simulink model "Simple_Variable_PID_KNN_gain_selector"  (R2020a)
settings: Solver=VariableStepAuto  StartTime=0.0  StopTime=0.08  RelTol=1e-3
undefined symbols (not defined in the file): Ion, Lithium
libraries: powerlib x15, simulink x3, powerlib_meascontrol x3, eeStairGenerator x3, electricdrivelib x1, re_lib x1
settings Model: Creator=Javier  LastModifiedBy=Javier

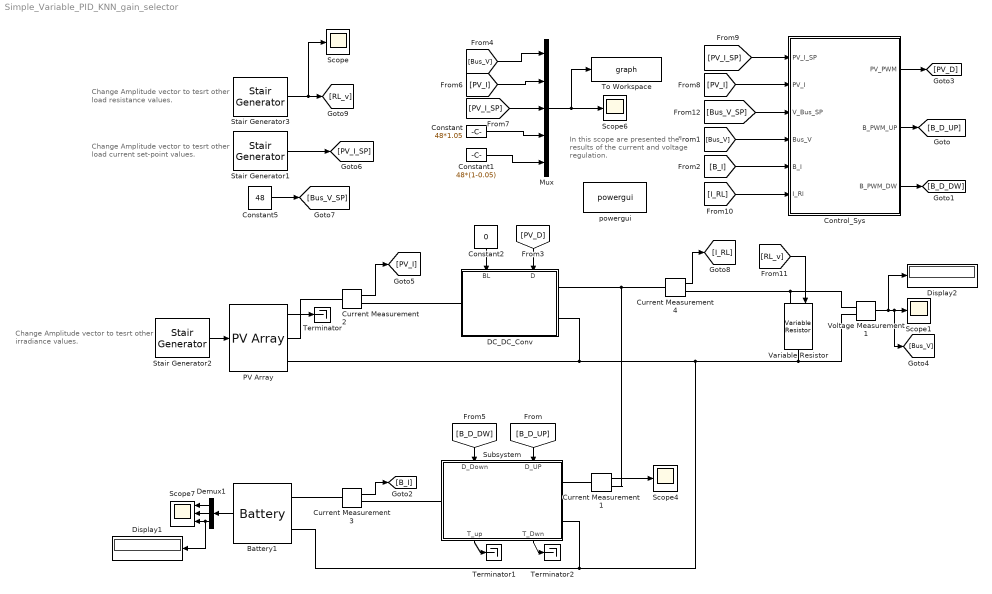
== system Simple_Variable_PID_KNN_gain_selector ==
  note: In this scope are presented the
      | results of the current and voltage
      | regulation.
  note: Change Amplitude vector to tesrt other
      | load resistance values.
  note: Change Amplitude vector to tesrt other
      | load current set-point values.
  note: Change Amplitude vector to tesrt other
      | irradiance values.
  Battery1 : electricdrivelib/Extra Sources/Battery  BatType=Lithium-Ion  ShowTempParam=off  ThermalPreset=no  ShowAgeParam=off  NomV=38.4  NomQ=2500  SOC=60  Batt_Tr=30  PresetModel=on  MaxQ=2500  MinV=28.8  FullV=44.6971  Dis_rate=1086.9565  R=0.0001536  Normal_OP=2260.8696  expZone="[41.48682      122.8261]"  current=[6.5 13 32.5]  Units=Time  Tci=20  NomT=20  T2=-30  MaxQ2=4.8  FullV2=7.1  Normal_OP2=5.655  expZone2="[6.58           1]"  Rca=0.6  ti=2000  Dp=0  Neq0=0  Tsim=1e6  Ta1=25  Qeol=5.4*0.9  Reol=0.013333*1.2  Char_age=[2.3478, 3]  Dis_age=[2.3478, 10]  N1=1500  N2=10500  N3=1000  N4=1400  Ta2=45  N5=950
  Constant : Constant  Value=48*1.05
  Constant1 : Constant  Value=48*(1-0.05)
  Constant2 : Constant  Value=0
  Constant5 : Constant  Value=48
  Control_Sys : Subsystem
  Current Measurement{1..4} (4 alike) : powerlib/Measurements/Current Measurement  PhasorSimulation=off  OutputType=Complex  PSBequivalent=0
  DC_DC_Conv : Subsystem
      settings: PortSchema="{\"entries\":[{\"content\":{\"sides\":[{\"content\":{\"connectorIds\":[\"LConn1\"]},\"type\":\"ConnectorPlacement.EquallySpacedRectSide\",\"uuid\":\"00f7090b-60ae-413e-b809-f771630d6751\"},{\"content\":{\"connectorIds\":[\"RConn1\",\"RConn2\"],\"side\":\"RIGHT\"},\"type\":\"ConnectorPlacement.EquallySpacedRectSide\",\"uuid\":\"f0025ab7-a9d8-466a-8e23-704d013948c1\"},{\"content\":{\"connectorIds\":[\"In1\",\"In2\"],\"side\":\"TOP\"},\"type\":\"ConnectorPlacement.EquallySpacedRectSide\",\"uuid\":\"5a345099-75bf-400d-9bb3-22f689fa92ef\"}]},\"type\":\"ConnectorPlacement.EquallySpacedConnector\",\"uuid\":\"2e1b2c5d-1adb-4779-83d3-3c40793dd951\"}],\"packageUris\":[\"http://schema.mathworks.com/mf0/Connector/19700101\"],\"version\":\"1.0\"}"
  Demux1 : Demux  Outputs=3
  Display1 : Display
  Display2 : Display
  Mux : Mux  Inputs=5
  PV Array : re_lib/Solar/PV Array  Npar=7  Nser=1  PlotType=array @ 1000 W/m2 & specified temperatures  S_vec="[ 1000  500  100 ]"  Temp_C_vec="[ 45 25  ]"  ModuleName=LG Electronics LG300N1W-G3  PlotWhenSelected=off  Pm=302.72  Ncell=60  Voc=39.5  Isc=10.05  Vm=32  Im=9.46  beta_Voc_pc=-0.3  alpha_Isc_pc=0.03  beta_Voc=-0.1185  alpha_Isc=0.003015  IL=10.0926  I0=3.3235e-11  nI=0.96984  Rsh=212.8143  Rs=0.31448  RobustModel=on  RobustCellTemperature=25  BAL=on  Tc=1e-7  Tfilter=1e-8
  Scope{,1,4,6} (4 alike) : Scope
  Scope7 : Scope  NumInputPorts=3
  Stair Generator1 : eeStairGenerator/Stair Generator  LabelModeActiveChoice=Discrete  TimeInput=[0 1 2 3 4 5 6]*0.01  AmplitudeInput=[0 3.323 6.645 49.65 23.28 6.645 0]  SampleTime=1/(1000e3)  RepeatPattern=off  OutDataTypeStr=double
      settings: SourceProductBaseCode=PS
  Stair Generator2 : eeStairGenerator/Stair Generator  LabelModeActiveChoice=Discrete  TimeInput=[0 1 2 3 4 5 6]*0.01  AmplitudeInput=[0 50 100 750 350 100 0]  SampleTime=1/(1000e3)  RepeatPattern=off  OutDataTypeStr=double
      settings: SourceProductBaseCode=PS
  Stair Generator3 : eeStairGenerator/Stair Generator  LabelModeActiveChoice=Discrete  TimeInput=[0 1 2 3 4 5 6]*0.01  AmplitudeInput=[10 5 1 10 20 20 20]  SampleTime=1/(1000e3)  RepeatPattern=off  OutDataTypeStr=double
      settings: SourceProductBaseCode=PS
  Subsystem : Subsystem
      settings: PortSchema="{\"entries\":[{\"content\":{\"sides\":[{\"content\":{\"connectorIds\":[\"LConn1\"]},\"type\":\"ConnectorPlacement.EquallySpacedRectSide\",\"uuid\":\"a9530ab3-8980-4dba-8483-d408c1c24a59\"},{\"content\":{\"connectorIds\":[\"RConn1\",\"RConn2\"],\"side\":\"RIGHT\"},\"type\":\"ConnectorPlacement.EquallySpacedRectSide\",\"uuid\":\"f691113d-6eb3-43ec-a6a4-3d8fb6884df6\"},{\"content\":{\"connectorIds\":[\"In1\",\"In2\"],\"side\":\"TOP\"},\"type\":\"ConnectorPlacement.EquallySpacedRectSide\",\"uuid\":\"a9eb11b6-05d7-4dbc-be9d-a17fd8550bb3\"},{\"content\":{\"connectorIds\":[\"Out1\",\"Out2\"],\"side\":\"BOTTOM\"},\"type\":\"ConnectorPlacement.EquallySpacedRectSide\",\"uuid\":\"90c7147c-e357-433a-9063-3b2a71587c45\"}]},\"type\":\"ConnectorPlacement.EquallySpacedConnector\",\"uuid\":\"b290d60f-d8ab-41f4-904b-2a909013e95d\"}],\"packageUris\":[\"http://schema.mathworks.com/mf0/Connector/19700101\"],\"version\":\"1.0\"}"
  Terminator : Terminator
  Terminator1 : Terminator
  Terminator2 : Terminator
  To Workspace : ToWorkspace  VariableName=graph  SaveFormat=Timeseries  SampleTime=-1
  Variable Resistor : powerlib/Elements/Variable Resistor  Rabsmin=1e-3
      settings: SourceProductBaseCode=PS
  Voltage Measurement1 : powerlib/Measurements/Voltage Measurement  PhasorSimulation=off  OutputType=Complex  PSBequivalent=0
  powergui : powerlib/powergui  Priority=1  SimulationMode=Discrete  SampleTime=1/(1000e3)  frequency=60  Iterations=50  frequencyindice=0  Pbase=100e6  ErrMax=1e-4  UnitsV=kV  UnitsW=MW  buscounter=0  FunctionMessages=off  echomessages=off  EnableUseOfTLC=off  CurrentSourceSwitches=off  DisableSnubberDevices=off  DisableRonSwitches=off  DisableVfSwitches=off  DisplayEquations=off  AutomaticDiscreteSolvers=off  SolverType=Tustin/Backward Euler (TBE)  Interpol=off  ExternalGateDelay=off  methode=off  Ts=100  x0status=blocks  SPID=on  SwTol=0  HookPort=off  NonlinearTolerance=1e-4  nMaxIteration=100  ContinueOnMaxIteration=off  RestoreLinks=warning  ResistiveCurrentMeasurement=off  Frange=[0:2:500]  Ylog=off  Xlog=on  ShowGrid=off  save=off  variable=ZData  structure=0  ZoomFFT=off  StartTime=0.0  cycles=1  DisplayStyle=1  fundamental=60  FreqAxis=off  MaxFrequency=1000  frequencyindicesteady=1  RmsSteady=1  display=off
  wires:
  Current Measurement2/1 -> [PV_I]
  Mux/1 -> To Workspace/1, Scope6/1
  Constant2/1 -> DC_DC_Conv/1(BL)
  Demux1/2 -> Scope7/2
  Demux1/3 -> Display1/1, Scope7/3
  Demux1/1 -> Scope7/1
  Battery1/1 -> Demux1/1
  Voltage Measurement1/1 -> [Bus_V], Scope1/1, Display2/1
  Current Measurement3/1 -> [B_I]
  [Bus_V] -> Mux/1
  [PV_I] -> Mux/2
  [PV_I_SP] -> Mux/3
  Control_Sys/2(B_PWM_UP) -> [B_D_UP]
  Control_Sys/3(B_PWM_DW) -> [B_D_DW]
  Constant5/1 -> [Bus_V_SP]
  [B_I] -> Control_Sys/5(B_I)
  Control_Sys/1(PV_PWM) -> [PV_D]
  [PV_D] -> DC_DC_Conv/2(D)
  Stair Generator1/1 -> [PV_I_SP]
  [B_D_DW] -> Subsystem/1(D_Down)
  [B_D_UP] -> Subsystem/2(D_UP)
  Current Measurement1/1 -> Scope4/1
  [PV_I_SP] -> Control_Sys/1(PV_I_SP)
  [PV_I] -> Control_Sys/2(PV_I)
  [Bus_V_SP] -> Control_Sys/3(V_Bus_SP)
  [Bus_V] -> Control_Sys/4(Bus_V)
  PV Array/1 -> Terminator/1
  Subsystem/2(T_Dwn) -> Terminator2/1
  Subsystem/1(T_up) -> Terminator1/1
  Current Measurement4/1 -> [I_RL]
  [I_RL] -> Control_Sys/6(I_Rl)
  Stair Generator2/1 -> PV Array/1
  Constant/1 -> Mux/4
  Constant1/1 -> Mux/5
  Stair Generator3/1 -> Scope/1, [RL_v]
  [RL_v] -> Variable Resistor/1
  connections:
  Current Measurement4/RConn1 -- Variable Resistor/LConn1 -- Voltage Measurement1/LConn1
  Subsystem/RConn2 -- Battery1/LConn2 -- DC_DC_Conv/RConn2 -- PV Array/RConn2 -- Variable Resistor/RConn1 -- Voltage Measurement1/LConn2
  Current Measurement2/RConn1 -- DC_DC_Conv/LConn1
  Current Measurement2/LConn1 -- PV Array/RConn1
  Current Measurement3/LConn1 -- Battery1/LConn1
  Current Measurement1/LConn1 -- Subsystem/RConn1
  Current Measurement3/RConn1 -- Subsystem/LConn1
  Current Measurement1/RConn1 -- Current Measurement4/LConn1 -- DC_DC_Conv/RConn1

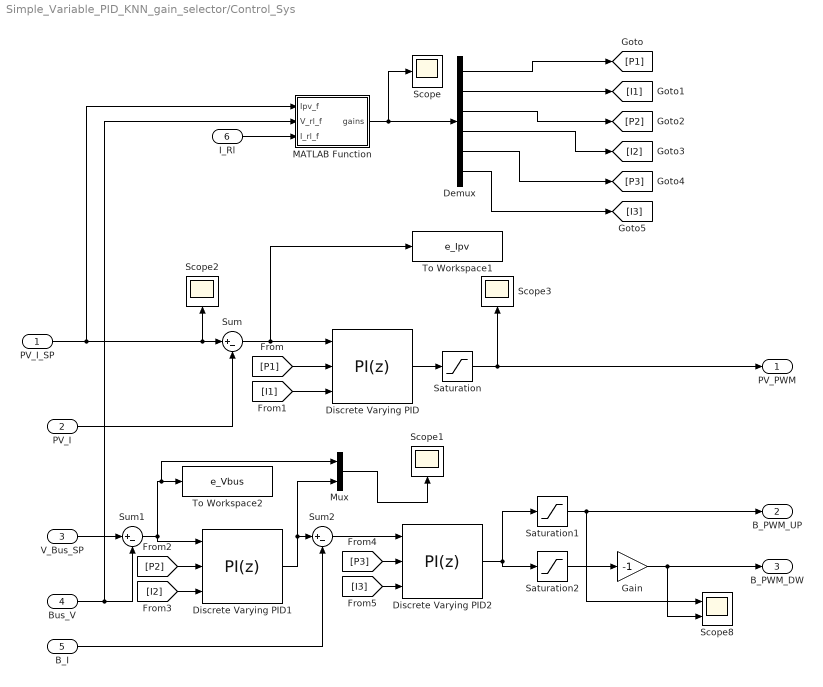
== system Simple_Variable_PID_KNN_gain_selector/Control_Sys ==
  PV_I_SP : Inport
  PV_I : Inport  Port=2
  V_Bus_SP : Inport  Port=3
  Bus_V : Inport  Port=4
  B_I : Inport  Port=5
  I_Rl : Inport  Port=6
  Demux : Demux  Outputs=6
  Discrete Varying PID : simulink/Continuous/PID Controller  Controller=PI  Form=Parallel  TimeDomain=Discrete-time  UseExternalTs=off  SampleTime=1/500e3  IntegratorMethod=Forward Euler  FilterMethod=Forward Euler  ControllerParametersSource=external  P=1  I=1  D=0  UseFilter=on  N=100  TunerSelectOption=Transfer Function Based (PID Tuner App)  InitialConditionSource=internal  InitialConditionForIntegrator=0  InitialConditionForFilter=0  DifferentiatorICPrevScaledInput=0  ExternalReset=none  TrackingMode=off  Kt=1  LimitOutput=on  UpperSaturationLimit=1  LowerSaturationLimit=-1  LinearizeAsGain=on  AntiWindupMode=none  Kb=1  POutMin=[]  POutMax=[]  IOutMin=[]  IOutMax=[]  DOutMin=[]  DOutMax=[]  NOutMin=[]  NOutMax=[]  SumOutMin=[]  SumOutMax=[]  SaturationOutMin=[]  SaturationOutMax=[]  PParamMin=[]  PParamMax=[]  IParamMin=[]  IParamMax=[]  DParamMin=[]  DParamMax=[]  NParamMin=[]  NParamMax=[]  KbParamMin=[]  KbParamMax=[]  KtParamMin=[]  KtParamMax=[]  KbOutMin=[]  KbOutMax=[]  KtOutMin=[]  KtOutMax=[]  IntegratorOutMin=[]  IntegratorOutMax=[]  FilterOutMin=[]  FilterOutMax=[]  SumI1OutMin=[]  SumI1OutMax=[]  SumI2OutMin=[]  SumI2OutMax=[]  SumI3OutMin=[]  SumI3OutMax=[]  SumI4OutMin=[]  SumI4OutMax=[]  SumDOutMin=[]  SumDOutMax=[]  DifferentiatorOutMin=[]  DifferentiatorOutMax=[]  FilterDiffOutCoefMin=[]  FilterDiffOutCoefMax=[]  ReciprocalOutMin=[]  ReciprocalOutMax=[]  SumDenOutMin=[]  SumDenOutMax=[]  SumNumOutMin=[]  SumNumOutMax=[]  DivideOutMin=[]  DivideOutMax=[]  UdiffTsProdOutMin=[]  UdiffTsProdOutMax=[]  NTsProdOutMin=[]  NTsProdOutMax=[]  UintegralTsProdOutMin=[]  UintegralTsProdOutMax=[]  UngainTsProdOutMin=[]  UngainTsProdOutMax=[]  IntegratorContinuousStateAttributes=''  IntegratorStateMustResolveToSignalObject=off  IntegratorRTWStateStorageClass=Auto  FilterContinuousStateAttributes=''  FilterStateMustResolveToSignalObject=off  FilterRTWStateStorageClass=Auto  ParallelPVariant=ExternalParameters  IdealPVariant=Disabled  IVariant=ExternalParameters  DVariant=Disabled  IntegratorVariant=Discrete  SatVariant=Enabled  AWVariant=Passthrough  PCopyVariant=Disabled  TRVariant=Disabled  FdbkBlocksVariant=Forward  IdealPFdbkVariant=Disabled  SatFdbkVariant=Disabled  DerivativeFilterVariant=Disabled  NVariant=Disabled  NCopyVariant=Disabled_SignalSpec  FilterICVariant=Disabled  IntegratorICVariant=InternalICs  ExternalResetVariant=Disabled  TRSumVariant=Passthrough  SumFdbkVariant=Disabled  SumVariant=Sum_PI  TsampFilterVariant=InternalTs  TsampNgainVariant=Passthrough  TsampIntegralVariant=Passthrough
  Discrete Varying PID1 : simulink/Continuous/PID Controller  Controller=PI  Form=Parallel  TimeDomain=Discrete-time  UseExternalTs=off  SampleTime=1/500e3  IntegratorMethod=Forward Euler  FilterMethod=Forward Euler  ControllerParametersSource=external  P=1  I=1  D=0  UseFilter=on  N=100  TunerSelectOption=Transfer Function Based (PID Tuner App)  InitialConditionSource=internal  InitialConditionForIntegrator=0  InitialConditionForFilter=0  DifferentiatorICPrevScaledInput=0  ExternalReset=none  TrackingMode=off  Kt=1  LimitOutput=off  UpperSaturationLimit=500  LowerSaturationLimit=-500  LinearizeAsGain=on  AntiWindupMode=none  Kb=1  POutMin=[]  POutMax=[]  IOutMin=[]  IOutMax=[]  DOutMin=[]  DOutMax=[]  NOutMin=[]  NOutMax=[]  SumOutMin=[]  SumOutMax=[]  SaturationOutMin=[]  SaturationOutMax=[]  PParamMin=[]  PParamMax=[]  IParamMin=[]  IParamMax=[]  DParamMin=[]  DParamMax=[]  NParamMin=[]  NParamMax=[]  KbParamMin=[]  KbParamMax=[]  KtParamMin=[]  KtParamMax=[]  KbOutMin=[]  KbOutMax=[]  KtOutMin=[]  KtOutMax=[]  IntegratorOutMin=[]  IntegratorOutMax=[]  FilterOutMin=[]  FilterOutMax=[]  SumI1OutMin=[]  SumI1OutMax=[]  SumI2OutMin=[]  SumI2OutMax=[]  SumI3OutMin=[]  SumI3OutMax=[]  SumI4OutMin=[]  SumI4OutMax=[]  SumDOutMin=[]  SumDOutMax=[]  DifferentiatorOutMin=[]  DifferentiatorOutMax=[]  FilterDiffOutCoefMin=[]  FilterDiffOutCoefMax=[]  ReciprocalOutMin=[]  ReciprocalOutMax=[]  SumDenOutMin=[]  SumDenOutMax=[]  SumNumOutMin=[]  SumNumOutMax=[]  DivideOutMin=[]  DivideOutMax=[]  UdiffTsProdOutMin=[]  UdiffTsProdOutMax=[]  NTsProdOutMin=[]  NTsProdOutMax=[]  UintegralTsProdOutMin=[]  UintegralTsProdOutMax=[]  UngainTsProdOutMin=[]  UngainTsProdOutMax=[]  IntegratorContinuousStateAttributes=''  IntegratorStateMustResolveToSignalObject=off  IntegratorRTWStateStorageClass=Auto  FilterContinuousStateAttributes=''  FilterStateMustResolveToSignalObject=off  FilterRTWStateStorageClass=Auto  ParallelPVariant=ExternalParameters  IdealPVariant=Disabled  IVariant=ExternalParameters  DVariant=Disabled  IntegratorVariant=Discrete  SatVariant=Disabled  AWVariant=Passthrough  PCopyVariant=Disabled  TRVariant=Disabled  FdbkBlocksVariant=Forward  IdealPFdbkVariant=Disabled  SatFdbkVariant=Disabled  DerivativeFilterVariant=Disabled  NVariant=Disabled  NCopyVariant=Disabled_SignalSpec  FilterICVariant=Disabled  IntegratorICVariant=InternalICs  ExternalResetVariant=Disabled  TRSumVariant=Passthrough  SumFdbkVariant=Disabled  SumVariant=Sum_PI  TsampFilterVariant=InternalTs  TsampNgainVariant=Passthrough  TsampIntegralVariant=Passthrough
  Discrete Varying PID2 : simulink/Continuous/PID Controller  Controller=PI  Form=Parallel  TimeDomain=Discrete-time  UseExternalTs=off  SampleTime=1/500e3  IntegratorMethod=Forward Euler  FilterMethod=Forward Euler  ControllerParametersSource=external  P=1  I=1  D=0  UseFilter=on  N=100  TunerSelectOption=Transfer Function Based (PID Tuner App)  InitialConditionSource=internal  InitialConditionForIntegrator=0  InitialConditionForFilter=0  DifferentiatorICPrevScaledInput=0  ExternalReset=none  TrackingMode=off  Kt=1  LimitOutput=on  UpperSaturationLimit=1  LowerSaturationLimit=-1  LinearizeAsGain=on  AntiWindupMode=none  Kb=1  POutMin=[]  POutMax=[]  IOutMin=[]  IOutMax=[]  DOutMin=[]  DOutMax=[]  NOutMin=[]  NOutMax=[]  SumOutMin=[]  SumOutMax=[]  SaturationOutMin=[]  SaturationOutMax=[]  PParamMin=[]  PParamMax=[]  IParamMin=[]  IParamMax=[]  DParamMin=[]  DParamMax=[]  NParamMin=[]  NParamMax=[]  KbParamMin=[]  KbParamMax=[]  KtParamMin=[]  KtParamMax=[]  KbOutMin=[]  KbOutMax=[]  KtOutMin=[]  KtOutMax=[]  IntegratorOutMin=[]  IntegratorOutMax=[]  FilterOutMin=[]  FilterOutMax=[]  SumI1OutMin=[]  SumI1OutMax=[]  SumI2OutMin=[]  SumI2OutMax=[]  SumI3OutMin=[]  SumI3OutMax=[]  SumI4OutMin=[]  SumI4OutMax=[]  SumDOutMin=[]  SumDOutMax=[]  DifferentiatorOutMin=[]  DifferentiatorOutMax=[]  FilterDiffOutCoefMin=[]  FilterDiffOutCoefMax=[]  ReciprocalOutMin=[]  ReciprocalOutMax=[]  SumDenOutMin=[]  SumDenOutMax=[]  SumNumOutMin=[]  SumNumOutMax=[]  DivideOutMin=[]  DivideOutMax=[]  UdiffTsProdOutMin=[]  UdiffTsProdOutMax=[]  NTsProdOutMin=[]  NTsProdOutMax=[]  UintegralTsProdOutMin=[]  UintegralTsProdOutMax=[]  UngainTsProdOutMin=[]  UngainTsProdOutMax=[]  IntegratorContinuousStateAttributes=''  IntegratorStateMustResolveToSignalObject=off  IntegratorRTWStateStorageClass=Auto  FilterContinuousStateAttributes=''  FilterStateMustResolveToSignalObject=off  FilterRTWStateStorageClass=Auto  ParallelPVariant=ExternalParameters  IdealPVariant=Disabled  IVariant=ExternalParameters  DVariant=Disabled  IntegratorVariant=Discrete  SatVariant=Enabled  AWVariant=Passthrough  PCopyVariant=Disabled  TRVariant=Disabled  FdbkBlocksVariant=Forward  IdealPFdbkVariant=Disabled  SatFdbkVariant=Disabled  DerivativeFilterVariant=Disabled  NVariant=Disabled  NCopyVariant=Disabled_SignalSpec  FilterICVariant=Disabled  IntegratorICVariant=InternalICs  ExternalResetVariant=Disabled  TRSumVariant=Passthrough  SumFdbkVariant=Disabled  SumVariant=Sum_PI  TsampFilterVariant=InternalTs  TsampNgainVariant=Passthrough  TsampIntegralVariant=Passthrough
  Gain : Gain  Gain=-1
  MATLAB Function : MATLAB Function  TreatAsAtomicUnit=on
  Mux : Mux  Inputs=2
  Saturation : Saturate  UpperLimit=1  LowerLimit=0
  Saturation1 : Saturate  UpperLimit=0.99  LowerLimit=0
  Saturation2 : Saturate  UpperLimit=0  LowerLimit=-0.99
  Scope{,1..3} (4 alike) : Scope
  Scope8 : Scope  NumInputPorts=2
  Sum : Sum  Inputs=|+-
  Sum1 : Sum  Inputs=|+-
  Sum2 : Sum  Inputs=|+-
  To Workspace1 : ToWorkspace  VariableName=e_Ipv  SaveFormat=Timeseries  SampleTime=-1
  To Workspace2 : ToWorkspace  VariableName=e_Vbus  SaveFormat=Timeseries  SampleTime=-1
  PV_PWM : Outport
  B_PWM_UP : Outport  Port=2
  B_PWM_DW : Outport  Port=3
  wires:
  Saturation2/1 -> Gain/1
  PV_I_SP/1 -> MATLAB Function/1(Ipv_f), Scope2/1, Sum/1
  PV_I/1 -> Sum/2
  Saturation/1 -> Scope3/1, PV_PWM/1
  Sum/1 -> Discrete Varying PID/1, To Workspace1/1
  Discrete Varying PID2/1 -> Saturation1/1, Saturation2/1
  Gain/1 -> B_PWM_DW/1, Scope8/2
  Saturation1/1 -> B_PWM_UP/1, Scope8/1
  B_I/1 -> Sum2/2
  Sum1/1 -> Discrete Varying PID1/1, Mux/1, To Workspace2/1
  V_Bus_SP/1 -> Sum1/1
  Bus_V/1 -> MATLAB Function/2(V_rl_f), Sum1/2
  I_Rl/1 -> MATLAB Function/3(I_rl_f)
  [P1] -> Discrete Varying PID/2
  [I1] -> Discrete Varying PID/3
  Discrete Varying PID/1 -> Saturation/1
  Discrete Varying PID1/1 -> Mux/2, Sum2/1
  [P2] -> Discrete Varying PID1/2
  [I2] -> Discrete Varying PID1/3
  Sum2/1 -> Discrete Varying PID2/1
  [P3] -> Discrete Varying PID2/2
  [I3] -> Discrete Varying PID2/3
  Mux/1 -> Scope1/1
  MATLAB Function/1(gains) -> Scope/1, Demux/1
  Demux/1 -> [P1]
  Demux/2 -> [I1]
  Demux/3 -> [P2]
  Demux/4 -> [I2]
  Demux/5 -> [P3]
  Demux/6 -> [I3]

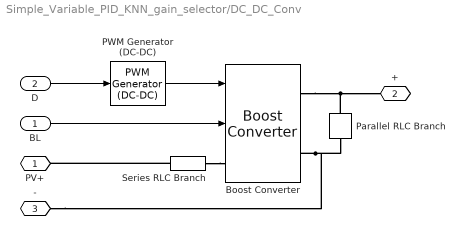
== system Simple_Variable_PID_KNN_gain_selector/DC_DC_Conv ==
  BL : Inport
  D : Inport  Port=2
  Boost Converter : powerlib/Power Electronics/Boost Converter  ModelType=Switching devices  Ron=1e-3  Rs=1e6  Cs=inf  Vforward=[0,0]  Ron_Diode=1e-3  Rs_Diode=1e6  Cs_Diode=inf  Vf_Diode=1e-3  Rs_CurrentSource=inf
      settings: SourceProductBaseCode=PS
  PWM Generator (DC-DC) : powerlib_meascontrol/Pulse & Signal Generators/PWM Generator (DC-DC)  Fsw=25e3  Ts=0
  Parallel RLC Branch : powerlib/Elements/Parallel RLC Branch  LConnTagsString=a  RConnTagsString=__new0  BranchType=C  Resistance=1e6  Inductance=1e-3  SetiL0=off  InitialCurrent=0  Capacitance=500e-6  Setx0=off  InitialVoltage=0  Measurements=None
  Series RLC Branch : powerlib/Elements/Series RLC Branch  LConnTagsString=__new0  RConnTagsString=__new0  BranchType=RL  Resistance=0.001  Inductance=96e-6  SetiL0=off  InitialCurrent=0  Capacitance=1e-6  Setx0=off  InitialVoltage=0  Measurements=None
  PV+ : PMIOPort  Side=Left
  + : PMIOPort  Port=2  Side=Right
  - : PMIOPort  Port=3  Side=Right
  wires:
  D/1 -> PWM Generator (DC-DC)/1
  PWM Generator (DC-DC)/1 -> Boost Converter/1
  BL/1 -> Boost Converter/2
  connections:
  Series RLC Branch/LConn1 -- PV+/RConn1
  Parallel RLC Branch/LConn1 -- Boost Converter/RConn1 -- +/RConn1
  Series RLC Branch/RConn1 -- Boost Converter/LConn1
  Boost Converter/RConn2 -- -/RConn1 -- Parallel RLC Branch/RConn1

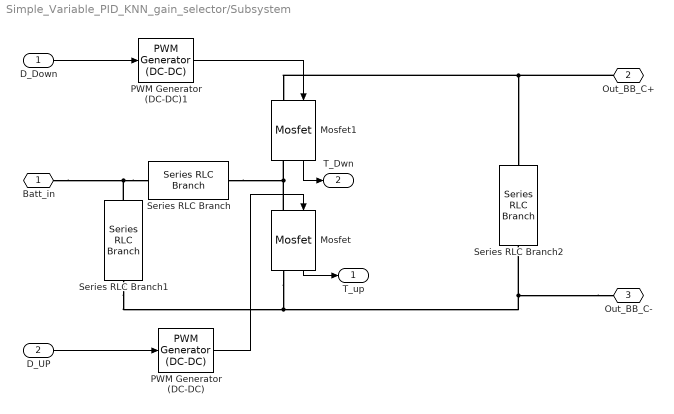
== system Simple_Variable_PID_KNN_gain_selector/Subsystem ==
  D_Down : Inport
  D_UP : Inport  Port=2
  Mosfet : powerlib/Power Electronics/Mosfet  Ron=0.1  Lon=0  Rd=0.01  Vfd=0  IC=0  Rs=1e5  Cs=inf  Measurements=on
  Mosfet1 : powerlib/Power Electronics/Mosfet  Ron=0.1  Lon=0  Rd=0.01  Vfd=0  IC=0  Rs=1e5  Cs=inf  Measurements=on
  PWM Generator (DC-DC) : powerlib_meascontrol/Pulse & Signal Generators/PWM Generator (DC-DC)  Fsw=25e3  Ts=0
  PWM Generator (DC-DC)1 : powerlib_meascontrol/Pulse & Signal Generators/PWM Generator (DC-DC)  Fsw=25e3  Ts=0
  Series RLC Branch : powerlib/Elements/Series RLC Branch  LConnTagsString=__new0  RConnTagsString=__new0  BranchType=L  Resistance=1  Inductance=5e-6  SetiL0=off  InitialCurrent=0  Capacitance=1e-6  Setx0=off  InitialVoltage=0  Measurements=None
  Series RLC Branch1 : powerlib/Elements/Series RLC Branch  LConnTagsString=__new0  RConnTagsString=__new0  BranchType=RC  Resistance=1  Inductance=1e-3  SetiL0=off  InitialCurrent=0  Capacitance=48e-6  Setx0=off  InitialVoltage=0  Measurements=None
  Series RLC Branch2 : powerlib/Elements/Series RLC Branch  LConnTagsString=__new0  RConnTagsString=__new0  BranchType=C  Resistance=1  Inductance=1e-3  SetiL0=off  InitialCurrent=0  Capacitance=48e-6  Setx0=off  InitialVoltage=0  Measurements=None
  Batt_in : PMIOPort  Side=Left
  Out_BB_C+ : PMIOPort  Port=2  Side=Right
  Out_BB_C- : PMIOPort  Port=3  Side=Right
  T_up : Outport
  T_Dwn : Outport  Port=2
  wires:
  PWM Generator (DC-DC)/1 -> Mosfet/1
  PWM Generator (DC-DC)1/1 -> Mosfet1/1
  Mosfet/1 -> T_up/1
  D_Down/1 -> PWM Generator (DC-DC)1/1
  Mosfet1/1 -> T_Dwn/1
  D_UP/1 -> PWM Generator (DC-DC)/1
  connections:
  Out_BB_C-/RConn1 -- Series RLC Branch2/RConn1 -- Mosfet/RConn1 -- Series RLC Branch1/RConn1
  Series RLC Branch/LConn1 -- Batt_in/RConn1 -- Series RLC Branch1/LConn1
  Out_BB_C+/RConn1 -- Mosfet1/LConn1 -- Series RLC Branch2/LConn1
  Mosfet/LConn1 -- Series RLC Branch/RConn1 -- Mosfet1/RConn1

== matlab function Simple_Variable_PID_KNN_gain_selector/Control_Sys/MATLAB Function ==
  data: Ipv_f input; gains output; V_rl_f input; I_rl_f input
function gains = fcn(Ipv_f,V_rl_f, I_rl_f)
    if I_rl_f==0
        R=20;
    else
        R=V_rl_f/I_rl_f;
    end
    X=[66.22 33.22 6.645 66.22 33.22 6.645 6.645 33.22 66.22 66.22 33.22 6.645;...
    20 20 20 10 10 10 1 1 1 0.5 0.5 0.5]';
    n = knnsearch(X,[Ipv_f R]);
    switch n
        case 1
            gains=[163.7768	596.7455 103.1845 3000 0.01	402.3498];
        case 2
            gains=[495.4661	4974.1 32.6379 3000	0.01 1073];
        case 3
            gains=[140.068 545.8923 92.8314 4.166 0.01 36.8058];
        case 4
            gains=[480.2696	467.6542 122.3516 501.0607 59.466 8.5631];
        case 5
            gains=[1.7114 2516.2 85.2561 3000 0.01 138.5982];
        case 6
            gains=[2.864 2103.4 24.5788 2899.1 0.01 0.01]; %gains=[2.864 2103.4 85.2561 2899.1 0.01 0.01]
        case 7
            gains=[0.974 3000 0.01 2615.4 519.9616 708.6039];
        case 8
            gains=[1.7312 2997.9 43.2105 0.01 583.8314 949.8327];
        case 9
            gains=[486.0544 1605 48.7177 2994.3 770.1381 2521.9];
        case 10
            gains=[140.4828	255.1471 25.0894 2992 977.4486 1625.8];
        case 11
            gains=[498.7227 496.5164 10.6462 3000 795.451 1818.7];
        case 12
            gains=[117.7502 0.01 408.6782 1617 875.7 1104.6]; %gains=[117.7502 0.01 408.6782 1617 875.7 1104.6];
        otherwise
            gains=[163.7768	596.7455 103.1845 3000 0.01	402.3498];
    end
